simulink model "DeepLearningDataCreator"  (R2020b)
settings: Solver=VariableStepAuto  StartTime=0.0  StopTime=100  RelTol=1e-3
undefined symbols (not defined in the file): gray, InitalDroneXYZ, ts_camera
libraries: dspvision x3, simulink x1, sim3dcameralib x1, sim3dlib x1, uavsim3dlib x1
settings Model: DataDictionary=Dictionary.sldd  EnableAccessToBaseWorkspace=off  OrderedModelArguments=off  Creator=alons  LastModifiedBy=elbit

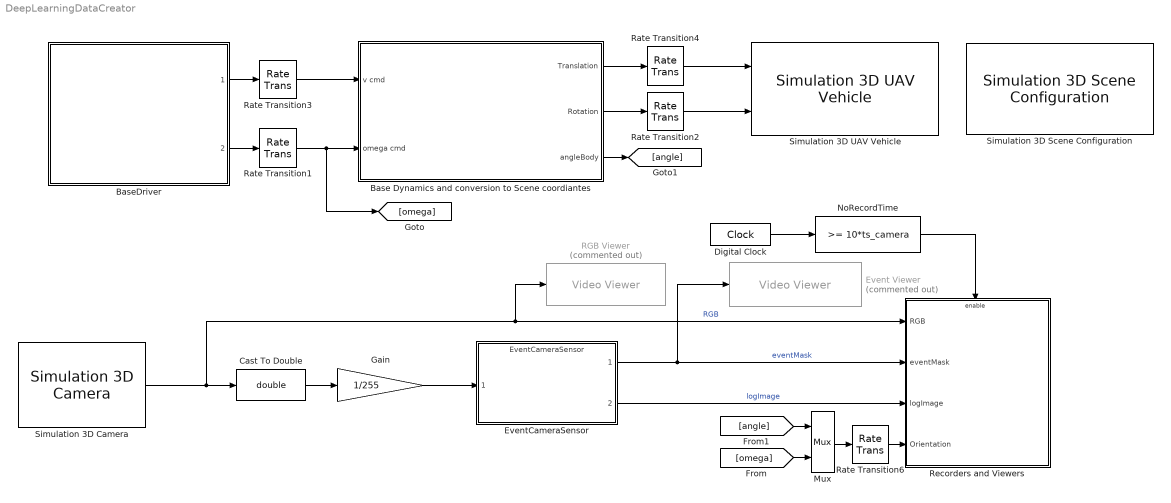
== system DeepLearningDataCreator ==
  Base Dynamics and conversion to Scene coordiantes : Subsystem  TreatAsAtomicUnit=on
  BaseDriver : Subsystem  TreatAsAtomicUnit=on  ReferencedSubsystem=BaseDriver
  Cast To Double : DataTypeConversion  OutDataTypeStr=double
  Digital Clock : DigitalClock  SampleTime=ts_camera
  Event Viewer : VideoViewer  Commented=on  colormapValue=gray(256)  FigPos=[728.2 681.2 676.8 413.6]
  EventCameraSensor : ModelReference  ModelNameDialog=EventCameraSensor  SimulationMode=Normal  ModelReferenceVersion=1.60
  Gain : Gain  Gain=1/255
  Mux : Mux  Inputs=2
  NoRecordTime : simulink/Logic and Bit Operations/Compare To Constant  relop=>=  const=10*ts_camera  OutDataTypeStr=boolean
  RGB Viewer : VideoViewer  Commented=on  FigPos=[669.8 730.8 733.6 478.4]
  Rate Transition1 : RateTransition  OutPortSampleTime=0
  Rate Transition2 : RateTransition
  Rate Transition3 : RateTransition  OutPortSampleTime=0
  Rate Transition4 : RateTransition
  Rate Transition6 : RateTransition  OutPortSampleTime=ts_camera
  Recorders and Viewers : Subsystem
  Simulation 3D Camera : sim3dcameralib/Simulation 3D Camera  Priority=1  sensorTag=Sim3dSensor2  sensorId=2  sensorName=Sim3dSensor2  vehTagList={'Drone';'Scene Origin';'SimulinkVehicle1'}  vehTag=Drone  mountLoc=Origin  offsetFlag=on  tmountOffset=[0.1, 0, 0]  rmountOffset=[0, 0, 0]  FocalLength=[1109, 1109]  OpticalCenter=[640, 360]  ImageSize=[720, 1280]  RadialDistortion=[0, 0]  TangentialDistortion=[0, 0]  SensorSkew=0  DepthOutportEnabled=off  SemanticOutportEnabled=off  TransformOutportEnabled=off  SampleTime=-1  mountPoint=[0.1 0 0]  mountOrientation=[0 0 0]  aMode=4  ID=2
      settings: SourceProductBaseCode=DR,UV,VE
  Simulation 3D Scene Configuration : sim3dlib/Simulation 3D Scene Configuration  Priority=0  ProjectFormat=Unreal Executable  SceneDesc=US city block  ProjectName=MathWorks_Aerospace.exe  ScenePath=/Game/Maps/USCityBlock  vehTagList={'Drone';'Scene Origin'}  vehTag=Drone  OpVisEn=off  Ts=ts_camera  EnableWindow=off  sensorTag=MainCamera1  sensorId=1  sensorName=MainCamera1  mountLoc=Origin  offsetFlag=off  tmountOffset=[0, 0, 0]  rmountOffset=[0, 0, 0]  HorizontalResolution=1280  VerticalResolution=720  HorizontalFOV=60  mountPoint=[0 0 0]  mountOrientation=[0 0 0]  aMode=4  ID=1
      settings: SourceProductBaseCode=DR,UV,VE
  Simulation 3D UAV Vehicle : uavsim3dlib/Simulation 3D UAV Vehicle  Mesh=Quadrotor  Color=Black  ActorName=Drone  InitialTranslation=InitalDroneXYZ  InitialRotation=[0 0 0]  SampleTime=-1  ActorType=SimulinkVehicle  ID=C  aMode=4  ActorTag=Drone
      settings: SourceProductName=UAV Toolbox
  wires:
  Simulation 3D Camera/1 -> RGB Viewer/1, Recorders and Viewers/1(RGB), Cast To Double/1  "RGB"
  Cast To Double/1 -> Gain/1
  Gain/1 -> EventCameraSensor/1
  BaseDriver/1 -> Rate Transition3/1
  Rate Transition4/1 -> Simulation 3D UAV Vehicle/1
  Rate Transition3/1 -> Base Dynamics and conversion to Scene coordiantes/1(v cmd)
  Base Dynamics and conversion to Scene coordiantes/1(Translation) -> Rate Transition4/1
  Base Dynamics and conversion to Scene coordiantes/2(Rotation) -> Rate Transition2/1
  EventCameraSensor/1 -> Event Viewer/1, Recorders and Viewers/2(eventMask)  "eventMask"
  EventCameraSensor/2 -> Recorders and Viewers/3(logImage)  "logImage"
  Mux/1 -> Rate Transition6/1
  Digital Clock/1 -> NoRecordTime/1
  [angle] -> Mux/1
  [omega] -> Mux/2
  NoRecordTime/1 -> Recorders and Viewers/Enable
  Rate Transition2/1 -> Simulation 3D UAV Vehicle/2
  Base Dynamics and conversion to Scene coordiantes/3(angleBody) -> [angle]
  Rate Transition6/1 -> Recorders and Viewers/4(Orientation)
  BaseDriver/2 -> Rate Transition1/1
  Rate Transition1/1 -> Base Dynamics and conversion to Scene coordiantes/2(omega cmd), [omega]

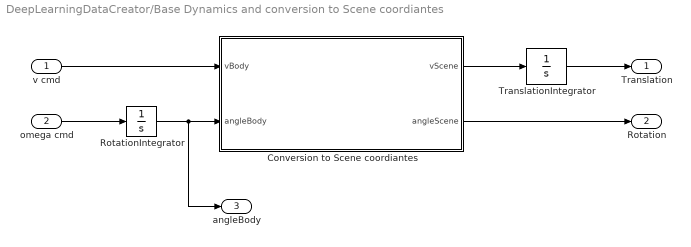
== system DeepLearningDataCreator/Base Dynamics and conversion to Scene coordiantes ==
  v cmd : Inport
  omega cmd : Inport  Port=2
  Conversion to Scene coordiantes : Subsystem
  RotationIntegrator : Integrator  InitialCondition="[0  0  0]"
  TranslationIntegrator : Integrator  InitialCondition=InitalDroneXYZ
  Translation : Outport
  Rotation : Outport  Port=2
  angleBody : Outport  Port=3
  wires:
  omega cmd/1 -> RotationIntegrator/1
  v cmd/1 -> Conversion to Scene coordiantes/1(vBody)
  RotationIntegrator/1 -> angleBody/1, Conversion to Scene coordiantes/2(angleBody)
  Conversion to Scene coordiantes/1(vScene) -> TranslationIntegrator/1
  Conversion to Scene coordiantes/2(angleScene) -> Rotation/1
  TranslationIntegrator/1 -> Translation/1

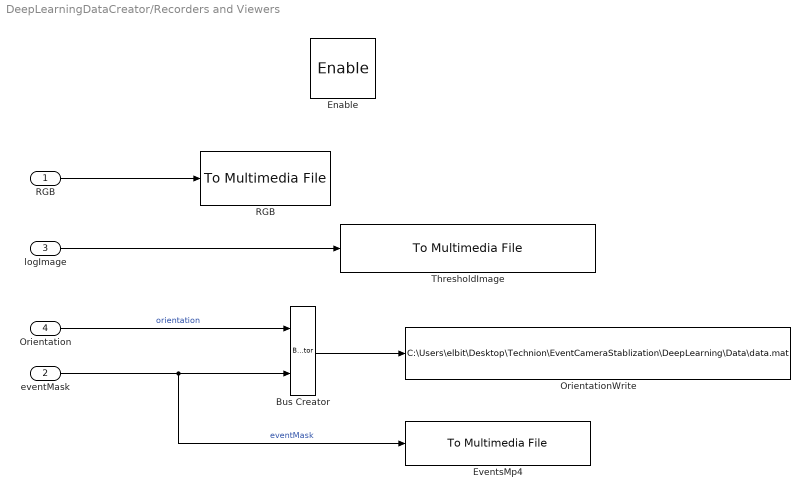
== system DeepLearningDataCreator/Recorders and Viewers ==
  RGB : Inport
  eventMask : Inport  Port=2
  logImage : Inport  Port=3
  Orientation : Inport  Port=4
  Enable : EnablePort
  Bus Creator : BusCreator  Inputs=2
  EventsMp4 : dspvision/To Multimedia File  outputFilename=C:\Users\elbit\Desktop\Technion\EventCameraStablization\DeepLearning\Data\eventMask.mp4  streamSelection=Video only  videoCompressor=None (uncompressed)  audioCompressor=None (uncompressed)  imagePorts=One multidimensional signal  fileType=MPEG4  audioDatatype=Determine from input data type  fourcc=RGB  videoQuality=100  mj2000CompFactor=10
  OrientationWrite : ToFile  Filename=C:\Users\elbit\Desktop\Technion\EventCameraStablization\DeepLearning\Data\data.mat  MatrixName=data  SaveFormat=Timeseries
  "RGB " : dspvision/To Multimedia File  outputFilename=C:\Users\elbit\Desktop\Technion\EventCameraStablization\DeepLearning\Data\RGB.mp4  streamSelection=Video only  videoCompressor=None (uncompressed)  audioCompressor=None (uncompressed)  imagePorts=One multidimensional signal  fileType=MPEG4  audioDatatype=Determine from input data type  fourcc=RGB  videoQuality=100  mj2000CompFactor=10
  ThresholdImage : dspvision/To Multimedia File  outputFilename=C:\Users\elbit\Desktop\Technion\EventCameraStablization\DeepLearning\Data\logImage.mp4  streamSelection=Video only  videoCompressor=None (uncompressed)  audioCompressor=None (uncompressed)  imagePorts=One multidimensional signal  fileType=MPEG4  audioDatatype=Determine from input data type  fourcc=RGB  videoQuality=100  mj2000CompFactor=10
  wires:
  RGB/1 -> "RGB "/1
  logImage/1 -> ThresholdImage/1
  Orientation/1 -> Bus Creator/1  "orientation"
  eventMask/1 -> EventsMp4/1, Bus Creator/2  "eventMask"
  Bus Creator/1 -> OrientationWrite/1

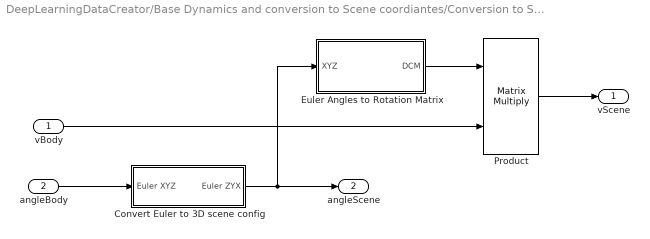
== system DeepLearningDataCreator/Base Dynamics and conversion to Scene coordiantes/Conversion to Scene coordiantes ==
  vBody : Inport
  angleBody : Inport  Port=2
  Convert Euler to 3D scene config : Subsystem
  Euler Angles to Rotation Matrix : Subsystem
  Product : Product  Multiplication=Matrix(*)
  vScene : Outport
  angleScene : Outport  Port=2
  wires:
  Product/1 -> vScene/1
  Convert Euler to 3D scene config/1(Euler ZYX) -> angleScene/1, Euler Angles to Rotation Matrix/1(XYZ)
  Euler Angles to Rotation Matrix/1(DCM) -> Product/1
  vBody/1 -> Product/2
  angleBody/1 -> Convert Euler to 3D scene config/1(Euler XYZ)

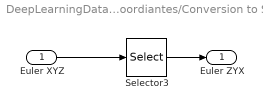
== system DeepLearningDataCreator/Base Dynamics and conversion to Scene coordiantes/Conversion to Scene coordiantes/Convert Euler to 3D scene config ==
  Euler XYZ : Inport
  Selector3 : Selector  InputPortWidth=3  IndexOptions=Index vector (dialog)  Indices=[3 2 1]  OutputSizes=1
  Euler ZYX : Outport
  wires:
  Selector3/1 -> Euler ZYX/1
  Euler XYZ/1 -> Selector3/1

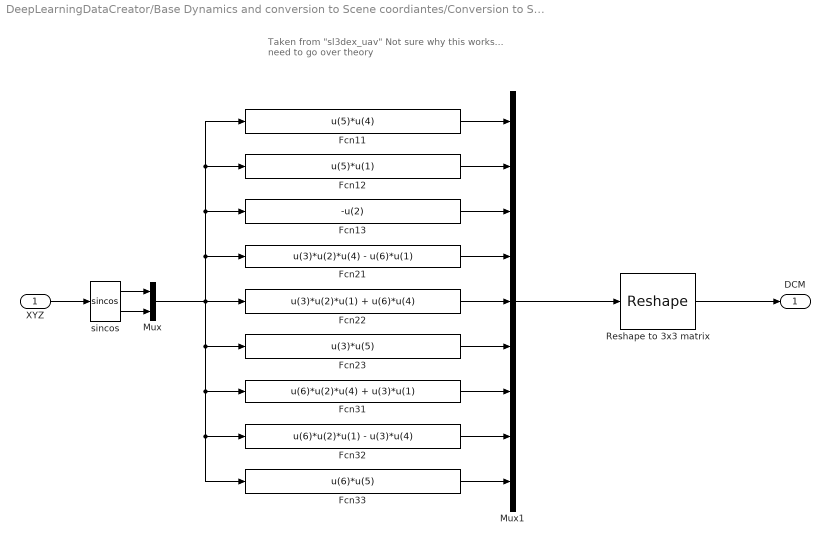
== system DeepLearningDataCreator/Base Dynamics and conversion to Scene coordiantes/Conversion to Scene coordiantes/Euler Angles to Rotation Matrix ==
  note: Taken from "sl3dex_uav"
      | Not sure why this works... need to go over theory
  XYZ : Inport
  Fcn11 : Fcn  Expr=u(5)*u(4)
  Fcn12 : Fcn  Expr=u(5)*u(1)
  Fcn13 : Fcn  Expr=-u(2)
  Fcn21 : Fcn  Expr=u(3)*u(2)*u(4) - u(6)*u(1)
  Fcn22 : Fcn  Expr=u(3)*u(2)*u(1) + u(6)*u(4)
  Fcn23 : Fcn  Expr=u(3)*u(5)
  Fcn31 : Fcn  Expr=u(6)*u(2)*u(4) + u(3)*u(1)
  Fcn32 : Fcn  Expr=u(6)*u(2)*u(1) - u(3)*u(4)
  Fcn33 : Fcn  Expr=u(6)*u(5)
  Mux : Mux  Inputs=2
  Mux1 : Mux  Inputs=9
  Reshape to 3x3 matrix : Reshape  OutputDimensionality=Customize  OutputDimensions=[3,3]
  sincos : Trigonometry  Operator=sincos
  DCM : Outport  Unit=1  PortDimensions=[3,3]  VectorParamsAs1DForOutWhenUnconnected=off
  wires:
  Mux/1 -> Fcn11/1, Fcn12/1, Fcn13/1, Fcn21/1, Fcn32/1, Fcn33/1, Fcn31/1, Fcn23/1, Fcn22/1
  sincos/2 -> Mux/2
  sincos/1 -> Mux/1
  XYZ/1 -> sincos/1
  Fcn11/1 -> Mux1/1
  Fcn12/1 -> Mux1/2
  Fcn13/1 -> Mux1/3
  Fcn21/1 -> Mux1/4
  Fcn22/1 -> Mux1/5
  Fcn23/1 -> Mux1/6
  Fcn31/1 -> Mux1/7
  Fcn32/1 -> Mux1/8
  Fcn33/1 -> Mux1/9
  Mux1/1 -> Reshape to 3x3 matrix/1
  Reshape to 3x3 matrix/1 -> DCM/1
